simulink library "environmentLib"  (R2020b)
settings: Solver=VariableStepAuto  StartTime=0.0  StopTime=10.0  RelTol=1e-3
undefined symbols (not defined in the file): initCond, km, s, vehicle, WMM2020
libraries: aerolibutil x2, FancyGravity x1, aerolibconvert2 x1, aerolibgravity2 x1, aerolibcelestial x1
settings Model: Creator=dbell44  LastModifiedBy=dbell44

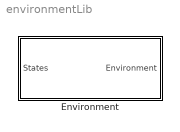
== system environmentLib ==
  Environment : Subsystem

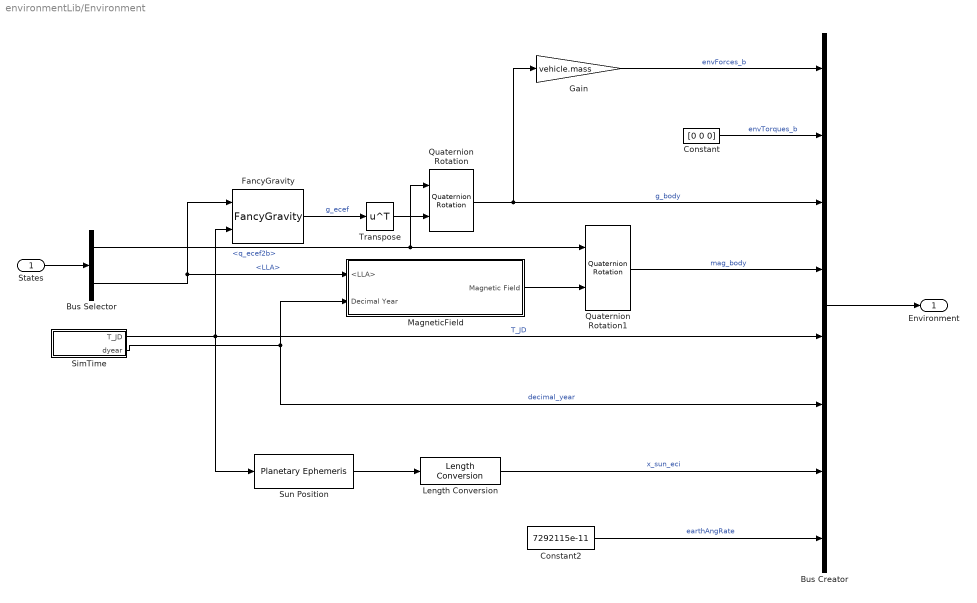
== system environmentLib/Environment ==
  States : Inport  OutDataTypeStr=Bus: States
  Bus Creator : BusCreator  Inputs=8
  Bus Selector : BusSelector  OutputSignals=q_ecef2b,LLA
  Constant : Constant  Value=[0 0 0]
  Constant2 : Constant  RequirementInfo={} %GIDa_a191e8b9_cb07_4d22_8813_52794fb76c2c  Value=7292115e-11
  FancyGravity : FancyGravity/FancyGravity  SystemSampleTime=-1  VariantActivationTime=update diagram  Latency=0  AutoFrameSizeCalculation=off
  Gain : Gain  Gain=vehicle.mass
  Length Conversion : aerolibconvert2/Length Conversion  IU=km  OU=m
  MagneticField : Subsystem
  Quaternion Rotation : aerolibutil/Quaternion Rotation
  Quaternion Rotation1 : aerolibutil/Quaternion Rotation
  SimTime : Subsystem
  Sun Position : aerolibcelestial/Planetary Ephemeris  kmflag=km,km/s  epochflag=Julian date  de=DE421  nCenter=Earth  nTarget=Sun  errorflag=Error  velflag=off
      settings: SourceProductBaseCode=AE
  Transpose : Math  Operator=transpose  SaturateOnIntegerOverflow=on
  Environment : Outport  OutDataTypeStr=Bus: Environment
  wires:
  Length Conversion/1 -> Bus Creator/7  "x_sun_eci"
  Gain/1 -> Bus Creator/1  "envForces_b"
  Bus Selector/1 -> Quaternion Rotation1/1, Quaternion Rotation/1  "<q_ecef2b>"
  Transpose/1 -> Quaternion Rotation/2
  Bus Selector/2 -> FancyGravity/1, MagneticField/1(<LLA>)  "<LLA>"
  MagneticField/1(Magnetic Field) -> Quaternion Rotation1/2
  Sun Position/1 -> Length Conversion/1
  SimTime/1(T_JD) -> FancyGravity/2, Bus Creator/5, Sun Position/1  "T_JD"
  Bus Creator/1 -> Environment/1
  Constant2/1 -> Bus Creator/8  "earthAngRate"
  States/1 -> Bus Selector/1
  SimTime/2(dyear) -> MagneticField/2(Decimal Year), Bus Creator/6  "decimal_year"
  FancyGravity/1 -> Transpose/1  "g_ecef"
  Quaternion Rotation/1 -> Gain/1, Bus Creator/3  "g_body"
  Quaternion Rotation1/1 -> Bus Creator/4  "mag_body"
  Constant/1 -> Bus Creator/2  "envTorques_b"

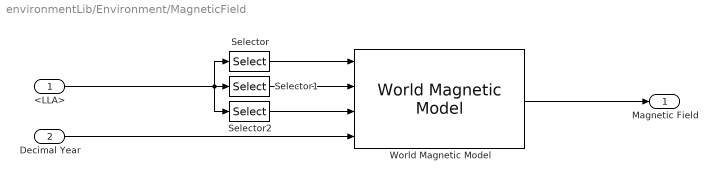
== system environmentLib/Environment/MagneticField ==
  <LLA> : Inport
  Decimal Year : Inport  Port=2
  Selector : Selector  InputPortWidth=3  IndexOptions=Index vector (dialog)  Indices=[3]  OutputSizes=1
  Selector1 : Selector  InputPortWidth=3  IndexOptions=Index vector (dialog)  Indices=[1]  OutputSizes=1
  Selector2 : Selector  InputPortWidth=3  IndexOptions=Index vector (dialog)  Indices=[2]  OutputSizes=1
  World Magnetic Model : aerolibgravity2/World Magnetic Model  model=WMM2020 (2020-2025)  customFile='WMM2020.COF'  units=Metric (MKS)  time_in=on  month=January  day=1  year=2020  action=Error  h_out=off  dec_out=off  inc_out=off  ti_out=off
      settings: SourceProductBaseCode=AE
  Magnetic Field : Outport
  wires:
  World Magnetic Model/1 -> Magnetic Field/1
  Selector/1 -> World Magnetic Model/1
  Decimal Year/1 -> World Magnetic Model/4
  Selector1/1 -> World Magnetic Model/2
  <LLA>/1 -> Selector2/1, Selector/1, Selector1/1
  Selector2/1 -> World Magnetic Model/3

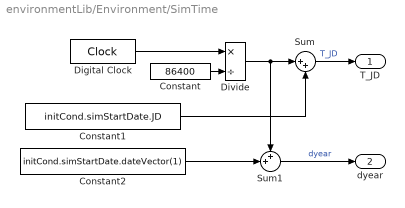
== system environmentLib/Environment/SimTime ==
  Constant : Constant  Value=86400
  Constant1 : Constant  Value=initCond.simStartDate.JD
  Constant2 : Constant  Value=initCond.simStartDate.dateVector(1)
  Digital Clock : DigitalClock
  Divide : Product  Inputs=*/
  Sum : Sum  Inputs=|++
  Sum1 : Sum  Inputs=++|
  T_JD : Outport
  dyear : Outport  Port=2
  wires:
  Sum/1 -> T_JD/1  "T_JD"
  Constant1/1 -> Sum/2
  Digital Clock/1 -> Divide/1
  Constant/1 -> Divide/2
  Divide/1 -> Sum/1, Sum1/1
  Constant2/1 -> Sum1/2
  Sum1/1 -> dyear/1  "dyear"
